simulink model "Exercise13"  (Simulink 7.2)
settings: Solver=ode45  StartTime=0.0  StopTime=10.0  RelTol=1e-3
undefined symbols (not defined in the file): des_figposition
libraries: simeventssink1 x2, simeventsprobes1 x2, simeventsgenerators1 x2, simulink x2, simeventsqueue1 x2, simeventsserver1 x2
settings Model: Creator=Inderjot  LastModifiedBy=Inderjot
settings SimEventsCC: propLogEventsScheduled=0  propLogEventsExecuted=0  propLogDepartureEvents=0  propDisplayEventCalendar=0  propDiagAttribOutput=1  propDiagFcnCallOutput=1  propDiagStatOutput=0

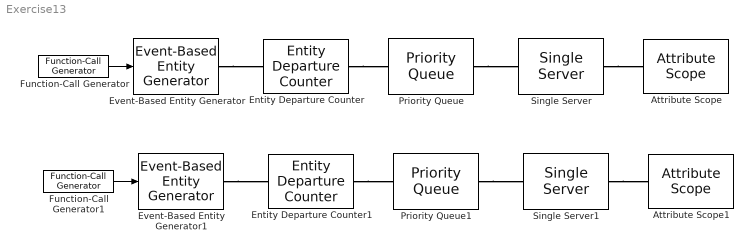
== system Exercise13 ==
  Attribute Scope : simeventssink1/Attribute Scope  Priority=1  SystemSampleTime=-1  PlotType=Stair  InputType=Attribute  NumInputs=1  AttributeNameY=Count  XInputOptionSignal=Event time  XInputOptionEntity=Event time  AttributeNameX=Count  EnableEntityOutport=on  XMin=0  XMax=10  XLimitExceededOption=Stretch axis limits  YLimitExceededOption=Stretch axis limits  AxisGrid=on  AxisLegend=off  LineDisables=""  LineColors=b  LineStyles=-  LineMarkers=.  OpenScopeAtSimStart=on  Title=""  YLabel=""  XLabel=Time  FigurePosition=des_figposition([5 25 25 25])  AxisZoom=off  DataStoreOption=Limited  DataPointsLimit=10000  StatNumberArrived=Off  ShowCountPlotted=off  ShowToolbar=on
      settings: YMin=0  YMax=10
  Attribute Scope1 : simeventssink1/Attribute Scope  Priority=1  SystemSampleTime=-1  PlotType=Stair  InputType=Attribute  NumInputs=1  AttributeNameY=Count  XInputOptionSignal=Event time  XInputOptionEntity=Event time  AttributeNameX=Count  EnableEntityOutport=on  XMin=0  XMax=10  XLimitExceededOption=Stretch axis limits  YLimitExceededOption=Stretch axis limits  AxisGrid=on  AxisLegend=off  LineDisables=""  LineColors=b  LineStyles=-  LineMarkers=.  OpenScopeAtSimStart=on  Title=""  YLabel=""  XLabel=Time  FigurePosition=des_figposition([5 25 25 25])  AxisZoom=off  DataStoreOption=Limited  DataPointsLimit=10000  StatNumberArrived=Off  ShowCountPlotted=off  ShowToolbar=on
      settings: YMin=0  YMax=10
  Entity Departure Counter : simeventsprobes1/Entity Departure Counter  Priority=1  SystemSampleTime=-1  NumberDepartedToSignal=Off  NumberDepartedToAttribute=On  NumberDepartedAttributeName=Count  CreateAttribute=on  CounterResetTypeOption=Off  CounterResetEdgeOption=Rising  SpecifyEventPriority=off  PriorityEntityCounterReset=1
  Entity Departure Counter1 : simeventsprobes1/Entity Departure Counter  Priority=1  SystemSampleTime=-1  NumberDepartedToSignal=Off  NumberDepartedToAttribute=On  NumberDepartedAttributeName=Count  CreateAttribute=on  CounterResetTypeOption=Off  CounterResetEdgeOption=Rising  SpecifyEventPriority=off  PriorityEntityCounterReset=1
  Event-Based Entity Generator : simeventsgenerators1/Entity Generators/Event-Based Entity Generator  Priority=1  DialogController=des_ddg_create  DialogControllerArgs=DataTag5  SystemSampleTime=-1  GenerateEntitiesUpon=Function call from port fcn  SignalEdgeType=Rising  SpecifyEventPriority=off  PriorityEntityGeneration=300  GenerateEntityAtSimulationStart=on  AllowBlocking=on  ResponseDuringBlockage=Discard generated entities  EntityType=Blank  StatNumberDeparted=Off  StatPendingEntity=Off  StatAverageIntergenerationTime=Off
  Event-Based Entity Generator1 : simeventsgenerators1/Entity Generators/Event-Based Entity Generator  Priority=1  DialogController=des_ddg_create  DialogControllerArgs=DataTag7  SystemSampleTime=-1  GenerateEntitiesUpon=Function call from port fcn  SignalEdgeType=Rising  SpecifyEventPriority=off  PriorityEntityGeneration=300  GenerateEntityAtSimulationStart=on  AllowBlocking=on  ResponseDuringBlockage=Discard generated entities  EntityType=Blank  StatNumberDeparted=Off  StatPendingEntity=Off  StatAverageIntergenerationTime=Off
  Function-Call Generator : simulink/Ports & Subsystems/Function-Call Generator  sample_time=10  numberOfIterations=9
  Function-Call Generator1 : simulink/Ports & Subsystems/Function-Call Generator  sample_time=10  numberOfIterations=9
  Priority Queue : simeventsqueue1/Priority Queue  Priority=1  SystemSampleTime=-1  Capacity=25  SortingAttributeName=Count  SortingDirection=Ascending  EnableTOPort=off  StatNumberDeparted=Off  StatNumberInBlock=Off  StatPendingEntity=Off  StatAverageWait=Off  StatAverageQueueLength=Off  StatNumberTimedout=Off
  Priority Queue1 : simeventsqueue1/Priority Queue  Priority=1  SystemSampleTime=-1  Capacity=25  SortingAttributeName=Count  SortingDirection=Descending  EnableTOPort=off  StatNumberDeparted=Off  StatNumberInBlock=Off  StatPendingEntity=Off  StatAverageWait=Off  StatAverageQueueLength=Off  StatNumberTimedout=Off
  Single Server : simeventsserver1/Single Server  Priority=1  SystemSampleTime=-1  ServiceTimeFrom=Dialog  ServiceTime=1  AttributeName=ServiceTime  PriorityServiceCompletion=500  PermitPreemption=off  SortingAttributeName=PriorityAttributeName  SortingDirection=Ascending  WriteToAttribute=off  ResidualAttributeName=ResidualServiceTime  CreateAttribute=on  EnableTOPort=off  StatNumberDeparted=Off  StatNumberInBlock=Off  StatNumberPreempted=Off  StatPendingEntity=Off  StatAverageWait=Off  StatUtilization=Off  StatNumberTimedout=Off
  Single Server1 : simeventsserver1/Single Server  Priority=1  SystemSampleTime=-1  ServiceTimeFrom=Dialog  ServiceTime=1  AttributeName=ServiceTime  PriorityServiceCompletion=500  PermitPreemption=off  SortingAttributeName=PriorityAttributeName  SortingDirection=Ascending  WriteToAttribute=off  ResidualAttributeName=ResidualServiceTime  CreateAttribute=on  EnableTOPort=off  StatNumberDeparted=Off  StatNumberInBlock=Off  StatNumberPreempted=Off  StatPendingEntity=Off  StatAverageWait=Off  StatUtilization=Off  StatNumberTimedout=Off
  wires:
  Function-Call Generator/1 -> Event-Based Entity Generator/1
  Function-Call Generator1/1 -> Event-Based Entity Generator1/1
  connections:
  Event-Based Entity Generator/RConn1 -- Entity Departure Counter/LConn1
  Entity Departure Counter/RConn1 -- Priority Queue/LConn1
  Priority Queue/RConn1 -- Single Server/LConn1
  Single Server/RConn1 -- Attribute Scope/LConn1
  Event-Based Entity Generator1/RConn1 -- Entity Departure Counter1/LConn1
  Single Server1/RConn1 -- Attribute Scope1/LConn1
  Entity Departure Counter1/RConn1 -- Priority Queue1/LConn1
  Priority Queue1/RConn1 -- Single Server1/LConn1
